simulink model "Simulate_ClassicalGAN"  (Simulink 10.2)
settings: Solver=ode45  StartTime=0.0  StopTime=60  RelTol=1e-3  EnableMultiTasking=on
libraries: fuzblock x2, slpidlib x2
settings Model: Creator=Administrator  LastModifiedBy=hunter
settings SolverCC: ZeroCrossControl=DisableAll
settings DataIOCC: LimitDataPoints=on
settings OptimizationCC: ExpressionDepthLimit=2147483647
settings DebuggingCC: SolverPrmCheckMsg=warning  StateNameClashWarn=warning

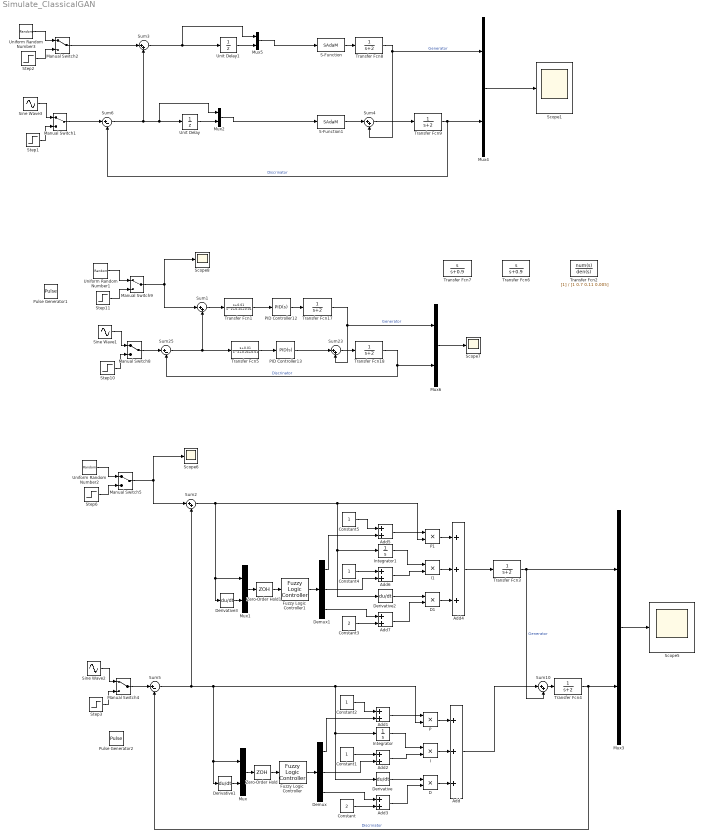
== system Simulate_ClassicalGAN ==
  Add : Sum  Inputs=+++
  Add{1..3,5..7} (6 alike) : Sum
  Add4 : Sum  Inputs=+++
  Constant : Constant  Value=2
  Constant{1..2,4..5} (4 alike) : Constant
  Constant3 : Constant  Value=2
  D : Product
  D1 : Product
  Demux : Demux  Outputs=3
  Demux1 : Demux  Outputs=3
  Derivative{,1..3} (4 alike) : Derivative
  Fuzzy Logic  Controller : fuzblock/Fuzzy Logic  Controller  FIS="\"fuzzypidcyq\""  OutputSampleNumber=1000  DataType=double  FuzzifiedInputs=off  RuleFiringStrengths=off  RuleOutputs=off  AggregatedOutputs=off  SimulateUsing=Interpreted execution  OutOfRangeInputValueMessage=warning  NoRuleFiredMessage=warning  EmptyOutputFuzzySetMessage=warning
  Fuzzy Logic  Controller1 : fuzblock/Fuzzy Logic  Controller  FIS="\"fuzzypidcyq\""  OutputSampleNumber=1000  DataType=double  FuzzifiedInputs=off  RuleFiringStrengths=off  RuleOutputs=off  AggregatedOutputs=off  SimulateUsing=Interpreted execution  OutOfRangeInputValueMessage=warning  NoRuleFiredMessage=warning  EmptyOutputFuzzySetMessage=warning
  I : Product
  I1 : Product
  Integrator : Integrator
  Integrator1 : Integrator
  Manual Switch{1..2,4..5,8..9} (6 alike) : ManualSwitch
  Mux{,1..6} (7 alike) : Mux  Inputs=2
  P : Product
  P1 : Product
  PID Controller12 : slpidlib/PID Controller  Controller=PID  Form=Parallel  TimeDomain=Continuous-time  UseExternalTs=off  SampleTime=-1  IntegratorMethod=Forward Euler  FilterMethod=Forward Euler  ControllerParametersSource=internal  P=1  I=0  D=0  UseFilter=on  N=100  TunerSelectOption=Transfer Function Based (PID Tuner App)  InitialConditionSource=internal  InitialConditionForIntegrator=0  InitialConditionForFilter=0  DifferentiatorICPrevScaledInput=0  ExternalReset=none  TrackingMode=off  Kt=1  LimitOutput=off  SatLimitsSource=internal  UpperSaturationLimit=inf  LowerSaturationLimit=-inf  LinearizeAsGain=on  AntiWindupMode=none  Kb=1  POutMin=[]  POutMax=[]  IOutMin=[]  IOutMax=[]  DOutMin=[]  DOutMax=[]  NOutMin=[]  NOutMax=[]  SumOutMin=[]  SumOutMax=[]  SaturationOutMin=[]  SaturationOutMax=[]  PParamMin=[]  PParamMax=[]  IParamMin=[]  IParamMax=[]  DParamMin=[]  DParamMax=[]  NParamMin=[]  NParamMax=[]  KbParamMin=[]  KbParamMax=[]  KtParamMin=[]  KtParamMax=[]  KbOutMin=[]  KbOutMax=[]  KtOutMin=[]  KtOutMax=[]  IntegratorOutMin=[]  IntegratorOutMax=[]  FilterOutMin=[]  FilterOutMax=[]  SumI1OutMin=[]  SumI1OutMax=[]  SumI2OutMin=[]  SumI2OutMax=[]  SumI3OutMin=[]  SumI3OutMax=[]  SumI4OutMin=[]  SumI4OutMax=[]  SumDOutMin=[]  SumDOutMax=[]  DifferentiatorOutMin=[]  DifferentiatorOutMax=[]  FilterDiffOutCoefMin=[]  FilterDiffOutCoefMax=[]  ReciprocalOutMin=[]  ReciprocalOutMax=[]  SumDenOutMin=[]  SumDenOutMax=[]  SumNumOutMin=[]  SumNumOutMax=[]  DivideOutMin=[]  DivideOutMax=[]  UdiffTsProdOutMin=[]  UdiffTsProdOutMax=[]  NTsProdOutMin=[]  NTsProdOutMax=[]  UintegralTsProdOutMin=[]  UintegralTsProdOutMax=[]  UngainTsProdOutMin=[]  UngainTsProdOutMax=[]  IntegratorContinuousStateAttributes=''  IntegratorStateMustResolveToSignalObject=off  IntegratorRTWStateStorageClass=Auto  FilterContinuousStateAttributes=''  FilterStateMustResolveToSignalObject=off  FilterRTWStateStorageClass=Auto  ParallelPVariant=InternalParameters  IdealPVariant=Disabled  IVariant=InternalParameters  DVariant=InternalParameters  IntegratorVariant=Continuous  SatVariant=Disabled  AWVariant=Passthrough  PCopyVariant=Disabled  TRVariant=Disabled  FdbkBlocksVariant=Forward  IdealPFdbkVariant=Disabled  SatFdbkVariant=Disabled  DerivativeFilterVariant=ContFilter  NVariant=InternalParameters  NCopyVariant=Disabled  FilterICVariant=InternalICsFilter  IntegratorICVariant=InternalICs  ExternalResetVariant=Disabled  TRSumVariant=Passthrough  SumFdbkVariant=Disabled  SumVariant=Sum_PID  TsampFilterVariant=InternalTs  TsampNgainVariant=Passthrough  TsampIntegralVariant=Passthrough  ExternalSaturationOutDataTypeStr=Inherit: Same as second input
  PID Controller13 : slpidlib/PID Controller  Controller=PID  Form=Parallel  TimeDomain=Continuous-time  UseExternalTs=off  SampleTime=-1  IntegratorMethod=Forward Euler  FilterMethod=Forward Euler  ControllerParametersSource=internal  P=1  I=0  D=0  UseFilter=on  N=100  TunerSelectOption=Transfer Function Based (PID Tuner App)  InitialConditionSource=internal  InitialConditionForIntegrator=0  InitialConditionForFilter=0  DifferentiatorICPrevScaledInput=0  ExternalReset=none  TrackingMode=off  Kt=1  LimitOutput=off  SatLimitsSource=internal  UpperSaturationLimit=inf  LowerSaturationLimit=-inf  LinearizeAsGain=on  AntiWindupMode=none  Kb=1  POutMin=[]  POutMax=[]  IOutMin=[]  IOutMax=[]  DOutMin=[]  DOutMax=[]  NOutMin=[]  NOutMax=[]  SumOutMin=[]  SumOutMax=[]  SaturationOutMin=[]  SaturationOutMax=[]  PParamMin=[]  PParamMax=[]  IParamMin=[]  IParamMax=[]  DParamMin=[]  DParamMax=[]  NParamMin=[]  NParamMax=[]  KbParamMin=[]  KbParamMax=[]  KtParamMin=[]  KtParamMax=[]  KbOutMin=[]  KbOutMax=[]  KtOutMin=[]  KtOutMax=[]  IntegratorOutMin=[]  IntegratorOutMax=[]  FilterOutMin=[]  FilterOutMax=[]  SumI1OutMin=[]  SumI1OutMax=[]  SumI2OutMin=[]  SumI2OutMax=[]  SumI3OutMin=[]  SumI3OutMax=[]  SumI4OutMin=[]  SumI4OutMax=[]  SumDOutMin=[]  SumDOutMax=[]  DifferentiatorOutMin=[]  DifferentiatorOutMax=[]  FilterDiffOutCoefMin=[]  FilterDiffOutCoefMax=[]  ReciprocalOutMin=[]  ReciprocalOutMax=[]  SumDenOutMin=[]  SumDenOutMax=[]  SumNumOutMin=[]  SumNumOutMax=[]  DivideOutMin=[]  DivideOutMax=[]  UdiffTsProdOutMin=[]  UdiffTsProdOutMax=[]  NTsProdOutMin=[]  NTsProdOutMax=[]  UintegralTsProdOutMin=[]  UintegralTsProdOutMax=[]  UngainTsProdOutMin=[]  UngainTsProdOutMax=[]  IntegratorContinuousStateAttributes=''  IntegratorStateMustResolveToSignalObject=off  IntegratorRTWStateStorageClass=Auto  FilterContinuousStateAttributes=''  FilterStateMustResolveToSignalObject=off  FilterRTWStateStorageClass=Auto  ParallelPVariant=InternalParameters  IdealPVariant=Disabled  IVariant=InternalParameters  DVariant=InternalParameters  IntegratorVariant=Continuous  SatVariant=Disabled  AWVariant=Passthrough  PCopyVariant=Disabled  TRVariant=Disabled  FdbkBlocksVariant=Forward  IdealPFdbkVariant=Disabled  SatFdbkVariant=Disabled  DerivativeFilterVariant=ContFilter  NVariant=InternalParameters  NCopyVariant=Disabled  FilterICVariant=InternalICsFilter  IntegratorICVariant=InternalICs  ExternalResetVariant=Disabled  TRSumVariant=Passthrough  SumFdbkVariant=Disabled  SumVariant=Sum_PID  TsampFilterVariant=InternalTs  TsampNgainVariant=Passthrough  TsampIntegralVariant=Passthrough  ExternalSaturationOutDataTypeStr=Inherit: Same as second input
  Pulse Generator1 : DiscretePulseGenerator  PulseType=Time based  Period=5  PulseWidth=50
  Pulse Generator2 : DiscretePulseGenerator  PulseType=Time based  Period=10  PulseWidth=50
  S-Function : S-Function  FunctionName=SAdaM  SFunctionDeploymentMode=off  EnableBusSupport=off
  S-Function1 : S-Function  FunctionName=SAdaM  SFunctionDeploymentMode=off  EnableBusSupport=off
  Scope{1,5..8} (5 alike) : Scope
  Sine Wave1 : Sin  SampleTime=0
  Sine Wave2 : Sin  SampleTime=0
  Sine Wave3 : Sin  SampleTime=0
  Step1 : Step  Time=0  SampleTime=0
  Step10 : Step  Time=0  SampleTime=0
  Step11 : Step  Time=10  SampleTime=0
  Step2 : Step  Time=10  SampleTime=0
  Step3 : Step  Time=0  SampleTime=0
  Step6 : Step  Time=10  SampleTime=0
  Sum{1..4,10,23} (6 alike) : Sum  Inputs=|++
  Sum25 : Sum  Inputs=|+-
  Sum5 : Sum  Inputs=|+-
  Sum6 : Sum  Inputs=|+-
  Transfer Fcn1 : TransferFcn  Numerator=[1 0.01]  Denominator=[1 0.2 0.01]
  Transfer Fcn{3..4,8..9,17..18} (6 alike) : TransferFcn  Denominator=[1 2]
  Transfer Fcn2 : TransferFcn  Denominator=[1 0.7 0.11 0.005]
  Transfer Fcn5 : TransferFcn  Numerator=[1 0.01]  Denominator=[1 0.2 0.01]
  Transfer Fcn6 : TransferFcn  Numerator=[1 0]  Denominator=[1 0.9]
  Transfer Fcn7 : TransferFcn  Numerator=[1 0]  Denominator=[1 0.9]
  Uniform Random Number1 : UniformRandomNumber  SampleTime=0.1
  Uniform Random Number2 : UniformRandomNumber  SampleTime=0.1
  Uniform Random Number3 : UniformRandomNumber  SampleTime=0.1
  Unit Delay : UnitDelay  SampleTime=-1  HasFrameUpgradeWarning=on
  Unit Delay1 : UnitDelay  SampleTime=-1  HasFrameUpgradeWarning=on
  Zero-Order Hold : ZeroOrderHold
  Zero-Order Hold1 : ZeroOrderHold
  wires:
  Manual Switch5/1 -> Sum2/1, Scope6/1
  Sine Wave2/1 -> Manual Switch4/1
  Transfer Fcn4/1 -> Sum5/2, Mux3/2  "Discrinator"
  Add/1 -> Sum10/1
  Add4/1 -> Transfer Fcn3/1
  Uniform Random Number2/1 -> Manual Switch5/1
  Mux3/1 -> Scope5/1
  Manual Switch4/1 -> Sum5/1
  Step3/1 -> Manual Switch4/2
  Transfer Fcn3/1 -> Sum10/2, Mux3/1  "Generator"
  Step6/1 -> Manual Switch5/2
  Sum10/1 -> Transfer Fcn4/1
  Demux1/2 -> Add6/2
  Derivative2/1 -> D1/1
  P1/1 -> Add4/1
  Constant4/1 -> Add6/1
  Add6/1 -> I1/2
  Add7/1 -> D1/2
  Constant3/1 -> Add7/2
  I1/1 -> Add4/2
  Integrator1/1 -> I1/1
  Sum2/1 -> Derivative2/1, Integrator1/1, P1/2, Derivative3/1, Mux1/1
  D1/1 -> Add4/3
  Add5/1 -> P1/1
  Demux1/3 -> Add7/1
  Constant5/1 -> Add5/1
  Demux1/1 -> Add5/2
  Derivative3/1 -> Mux1/2
  Demux/2 -> Add2/2
  Derivative/1 -> D/1
  P/1 -> Add/1
  Constant1/1 -> Add2/1
  Add2/1 -> I/2
  Add3/1 -> D/2
  Constant/1 -> Add3/2
  I/1 -> Add/2
  Integrator/1 -> I/1
  Sum5/1 -> Sum2/2, Derivative/1, Integrator/1, P/2, Derivative1/1, Mux/1
  D/1 -> Add/3
  Add1/1 -> P/1
  Demux/3 -> Add3/1
  Constant2/1 -> Add1/1
  Demux/1 -> Add1/2
  Derivative1/1 -> Mux/2
  Zero-Order Hold1/1 -> Fuzzy Logic  Controller1/1
  Zero-Order Hold/1 -> Fuzzy Logic  Controller/1
  Mux1/1 -> Zero-Order Hold1/1
  Mux/1 -> Zero-Order Hold/1
  Step10/1 -> Manual Switch8/2
  Manual Switch8/1 -> Sum25/1
  Step11/1 -> Manual Switch9/2
  Mux6/1 -> Scope7/1
  PID Controller12/1 -> Transfer Fcn17/1
  PID Controller13/1 -> Sum23/1
  Manual Switch9/1 -> Sum1/1, Scope8/1
  Sine Wave1/1 -> Manual Switch8/1
  Uniform Random Number1/1 -> Manual Switch9/1
  Transfer Fcn18/1 -> Mux6/2, Sum25/2  "Discrinator"
  Sum23/1 -> Transfer Fcn18/1
  Sum1/1 -> Transfer Fcn1/1
  Sum25/1 -> Transfer Fcn5/1, Sum1/2
  Transfer Fcn1/1 -> PID Controller12/1
  Transfer Fcn5/1 -> PID Controller13/1
  Transfer Fcn17/1 -> Mux6/1, Sum23/2  "Generator"
  S-Function1/1 -> Sum4/1
  Sum3/1 -> Mux5/1, Unit Delay1/1
  Unit Delay1/1 -> Mux5/2
  Mux5/1 -> S-Function/1
  Mux4/1 -> Scope1/1
  Transfer Fcn9/1 -> Mux4/2, Sum6/2  "Discrinator"
  Transfer Fcn8/1 -> Mux4/1, Sum4/2  "Generator"
  Sum6/1 -> Mux2/1, Unit Delay/1, Sum3/2
  Sum4/1 -> Transfer Fcn9/1
  S-Function/1 -> Transfer Fcn8/1
  Step2/1 -> Manual Switch2/2
  Uniform Random Number3/1 -> Manual Switch2/1
  Manual Switch2/1 -> Sum3/1
  Sine Wave3/1 -> Manual Switch1/1
  Manual Switch1/1 -> Sum6/1
  Step1/1 -> Manual Switch1/2
  Unit Delay/1 -> Mux2/2
  Mux2/1 -> S-Function1/1
  Fuzzy Logic  Controller1/1 -> Demux1/1
  Fuzzy Logic  Controller/1 -> Demux/1
